simulink subsystem "ControlPhase"  (R2023a)
settings: Solver=VariableStepAuto  StartTime=0.0  StopTime=10.0  RelTol=1e-3
libraries: simulink x9
settings Model: Creator=lukasz  LastModifiedBy=lukasz

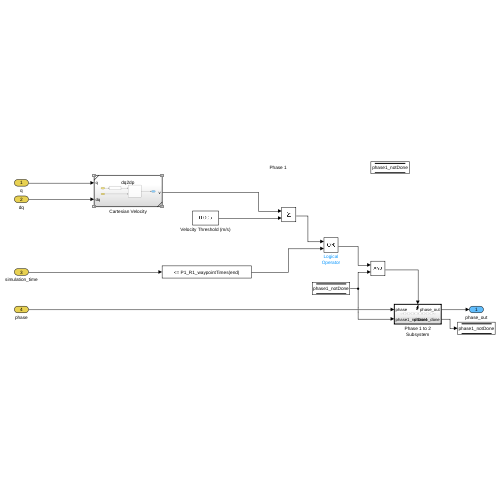
[thumbnail: Simulink's stored preview of the top-level diagram]
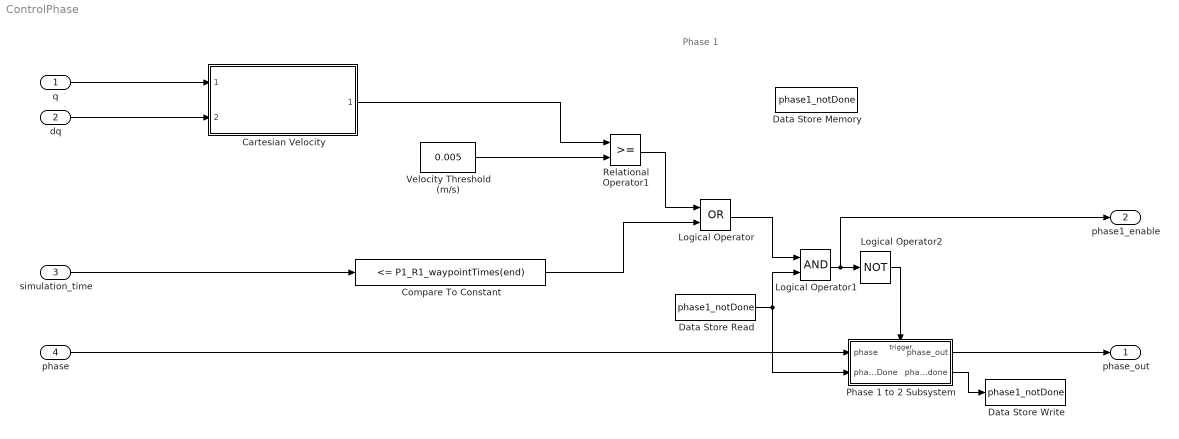
== system ControlPhase ==
  note: Phase 1
  q : Inport
  dq : Inport  Port=2
  simulation_time : Inport  Port=3
  phase : Inport  Port=4
  Cartesian Velocity : Subsystem  ReferencedSubsystem=dq2dp
  Compare To Constant : simulink/Logic and Bit Operations/Compare To Constant  relop=<=  const=P1_R1_waypointTimes(end)  OutDataTypeStr=boolean
  Data Store Memory : DataStoreMemory  DataStoreName=phase1_notDone  WriteAfterWriteMsg=warning  InitialValue=1  ShowAdditionalParam=off  OutDataTypeStr=boolean
  Data Store Read : DataStoreRead  DataStoreName=phase1_notDone  IndexOptions=Index vector (dialog)  Indices=1  OutputSizes=1
  Data Store Write : DataStoreWrite  DataStoreName=phase1_notDone  IndexOptions=Index vector (dialog)  Indices=1  OutputSizes=1
  Logical Operator : Logic  Operator=OR  AllPortsSameDT=off  OutDataTypeStr=boolean
  Logical Operator1 : Logic  AllPortsSameDT=off  OutDataTypeStr=boolean
  Logical Operator2 : Logic  Operator=NOT  AllPortsSameDT=off  OutDataTypeStr=boolean
  Phase 1 to 2 Subsystem : Subsystem  TreatAsAtomicUnit=on
  Relational Operator1 : RelationalOperator  OutDataTypeStr=boolean  RndMeth=Simplest  InputSameDT=off
  Velocity Threshold (m/s) : Constant  Value=0.005
  phase_out : Outport
  phase1_enable : Outport  Port=2
  wires:
  Velocity Threshold (m/s)/1 -> Relational Operator1/2
  Cartesian Velocity/1 -> Relational Operator1/1
  q/1 -> Cartesian Velocity/1
  dq/1 -> Cartesian Velocity/2
  Relational Operator1/1 -> Logical Operator/1
  Compare To Constant/1 -> Logical Operator/2
  Logical Operator/1 -> Logical Operator1/1
  Data Store Read/1 -> Phase 1 to 2 Subsystem/2(phase1_notDone), Logical Operator1/2
  Logical Operator1/1 -> Logical Operator2/1, phase1_enable/1
  phase/1 -> Phase 1 to 2 Subsystem/1(phase)
  Phase 1 to 2 Subsystem/1(phase_out) -> phase_out/1
  Phase 1 to 2 Subsystem/2(phase1_done) -> Data Store Write/1
  Logical Operator2/1 -> Phase 1 to 2 Subsystem/Trigger
  simulation_time/1 -> Compare To Constant/1

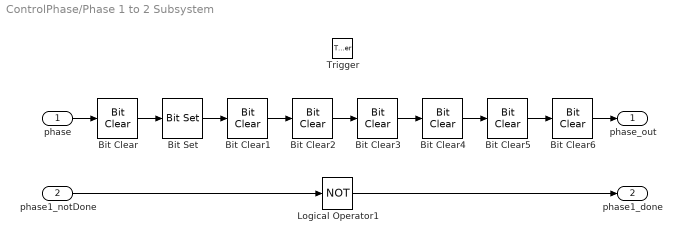
== system ControlPhase/Phase 1 to 2 Subsystem ==
  phase : Inport
  phase1_notDone : Inport  Port=2
  Trigger : TriggerPort  VariantControl=(inherit)
  Bit Clear : simulink/Logic and Bit Operations/Bit Clear  iBit=0
  Bit Clear1 : simulink/Logic and Bit Operations/Bit Clear  iBit=2
  Bit Clear2 : simulink/Logic and Bit Operations/Bit Clear  iBit=3
  Bit Clear3 : simulink/Logic and Bit Operations/Bit Clear  iBit=4
  Bit Clear4 : simulink/Logic and Bit Operations/Bit Clear  iBit=5
  Bit Clear5 : simulink/Logic and Bit Operations/Bit Clear  iBit=6
  Bit Clear6 : simulink/Logic and Bit Operations/Bit Clear  iBit=7
  Bit Set : simulink/Logic and Bit Operations/Bit Set  iBit=1
  Logical Operator1 : Logic  Operator=NOT  AllPortsSameDT=off  OutDataTypeStr=boolean
  phase_out : Outport
  phase1_done : Outport  Port=2
  wires:
  Bit Set/1 -> Bit Clear1/1
  phase/1 -> Bit Clear/1
  Bit Clear/1 -> Bit Set/1
  Bit Clear1/1 -> Bit Clear2/1
  Bit Clear2/1 -> Bit Clear3/1
  Bit Clear3/1 -> Bit Clear4/1
  Bit Clear4/1 -> Bit Clear5/1
  Bit Clear5/1 -> Bit Clear6/1
  Bit Clear6/1 -> phase_out/1
  phase1_notDone/1 -> Logical Operator1/1
  Logical Operator1/1 -> phase1_done/1
